simulink model "preLookupTestGen24"  (R2017b)
settings: Solver=FixedStepDiscrete  StartTime=0.0  StopTime=10.0  RelTol=1e-3
settings Model: Creator=ktrinh  LastModifiedBy=ktrinh
settings DebuggingCC: ParameterOverflowMsg=none

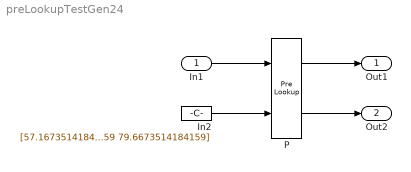
== system preLookupTestGen24 ==
  In1 : Inport  OutDataTypeStr=int16  PortDimensions=[2,3]
  In2 : Constant  Value=[57.1673514184159 58.6673514184159 60.1673514184159 61.6673514184159 63.1673514184159 64.6673514184159 66.1673514184159 67.6673514184159 69.1673514184159 70.6673514184159 72.1673514184159 73.6673514184159 75.1673514184159 76.6673514184159 78.1673514184159 79.6673514184159]
  P : PreLookup  BreakpointsDataSource=Input port  BreakpointsData=[10:10:110]  BeginIndexSearchUsingPreviousIndexResult=on  BreakpointDataTypeStr=int8  IndexDataTypeStr=int8  FractionDataTypeStr=double  RndMeth=Nearest
      settings: InputPortMap=u0,p1
  Out1 : Outport
  Out2 : Outport  Port=2
  wires:
  In1/1 -> P/1
  In2/1 -> P/2
  P/1 -> Out1/1
  P/2 -> Out2/1
